simulink model "FYP_Flywheel_Stage5_MODEL_v2"  (R2024a)
settings: Solver=ode45  StartTime=0.0  StopTime=18  RelTol=1e-3
values from neighbouring files (symbols this model uses):
  B = 1.0e-3    (= 0.001)    [FYP_Flywheel_Stage2_build.m]    (also in FYP_Flywheel_Stage3_DCServo_build.m; FYP_Flywheel_Stage4_v2_StableClosedLoop_build.m; FYP_Flywheel_Stage5_COMPLETE_v2.m)
  I_charge = 15    [FYP_Flywheel_Stage5_COMPLETE_v2.m]
  I_discharge = 15    [FYP_Flywheel_Stage5_COMPLETE_v2.m]
  Imax = 18    [FYP_Flywheel_Stage4_v2_StableClosedLoop_build.m]    (also in FYP_Flywheel_Stage5_COMPLETE_v2.m = 20)
  J_total = Jm + Jf    (= 0.51)    [FYP_Flywheel_Stage3_DCServo_build.m]    (also in FYP_Flywheel_Stage4_v2_StableClosedLoop_build.m; FYP_Flywheel_Stage5_COMPLETE_v2.m)
  Jf = 0.50    (= 0.5)    [FYP_Flywheel_Stage3_DCServo_build.m]    (also in FYP_Flywheel_Stage4_v2_StableClosedLoop_build.m; FYP_Flywheel_Stage5_COMPLETE_v2.m)
  Ke = 0.05    [FYP_Flywheel_Stage3_DCServo_build.m]    (also in FYP_Flywheel_Stage4_v2_StableClosedLoop_build.m; FYP_Flywheel_Stage5_COMPLETE_v2.m)
  Kp_current = 1.0    (= 1)    [FYP_Flywheel_Stage4_v2_StableClosedLoop_build.m]    (also in FYP_Flywheel_Stage5_COMPLETE_v2.m)
  Kt = 0.05    [FYP_Flywheel_Stage3_DCServo_build.m]    (also in FYP_Flywheel_Stage4_v2_StableClosedLoop_build.m; FYP_Flywheel_Stage5_COMPLETE_v2.m)
  L = 0.02    [FYP_Flywheel_Stage3_DCServo_build.m]    (also in FYP_Flywheel_Stage4_v2_StableClosedLoop_build.m; FYP_Flywheel_Stage5_COMPLETE_v2.m)
  omega0 = 2*pi*n0/60    (= 314.159265359)    [FYP_Flywheel_Stage1_build.m]    (also in FYP_Flywheel_Stage2_build.m; FYP_Flywheel_Stage3_DCServo_build.m; FYP_Flywheel_Stage4_v2_StableClosedLoop_build.m; FYP_Flywheel_Stage5_COMPLETE_v2.m)
  omega_max = 2*pi*n_max/60    (= 356.047167407)    [FYP_Flywheel_Stage2_build.m]    (also in FYP_Flywheel_Stage5_COMPLETE_v2.m = 329.867228627)
  omega_min = 2*pi*n_min/60    (= 293.215314335)    [FYP_Flywheel_Stage2_build.m]    (also in FYP_Flywheel_Stage5_COMPLETE_v2.m = 298.451302091)
  R = 0.8    [FYP_Flywheel_Stage3_DCServo_build.m]    (also in FYP_Flywheel_Stage4_v2_StableClosedLoop_build.m; FYP_Flywheel_Stage5_COMPLETE_v2.m)
  Tc = 0.05    [FYP_Flywheel_Stage2_build.m]    (also in FYP_Flywheel_Stage3_DCServo_build.m; FYP_Flywheel_Stage4_v2_StableClosedLoop_build.m; FYP_Flywheel_Stage5_COMPLETE_v2.m)
  Vmax = 60    [FYP_Flywheel_Stage4_v2_StableClosedLoop_build.m]    (also in FYP_Flywheel_Stage5_COMPLETE_v2.m)
settings Model: Creator=cheng  LastModifiedBy=cheng

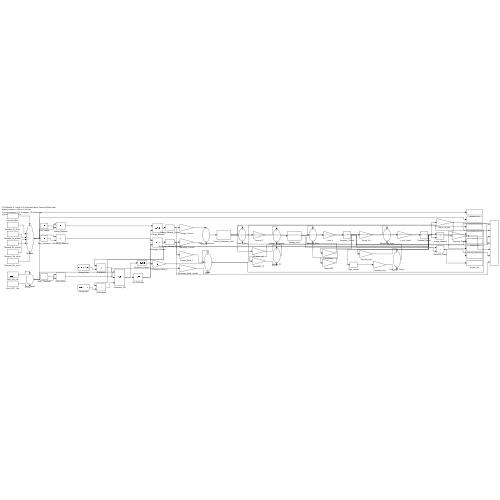
[thumbnail: Simulink's stored preview of the top-level diagram]
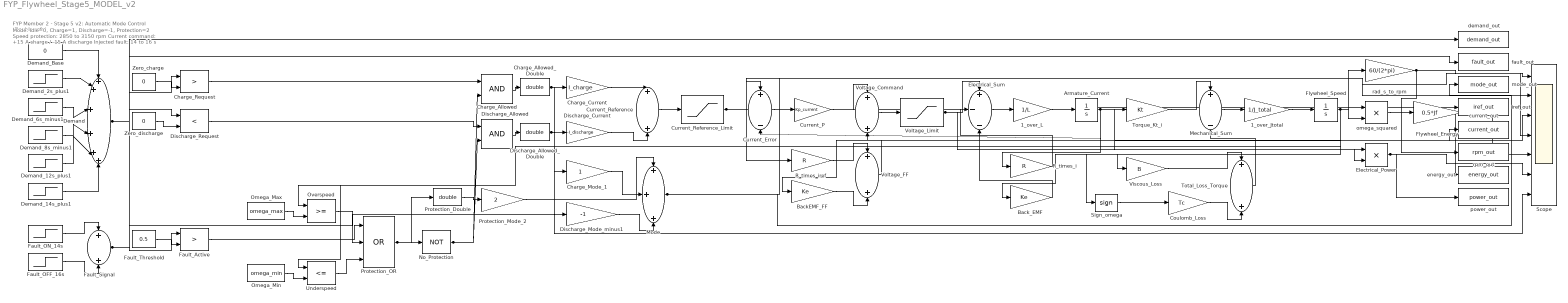
== system FYP_Flywheel_Stage5_MODEL_v2 ==
  note: FYP Member 2 - Stage 5 v2: Automatic Mode Control (Double-safe)
  note: Mode: Idle=0, Charge=1, Discharge=-1, Protection=2
      | Speed protection: 2850 to 3150 rpm
      | Current command: +15 A charge / -15 A discharge
      | Injected fault: 14 to 16 s
  1_over_Jtotal : Gain  Gain=1/J_total
  1_over_L : Gain  Gain=1/L
  Armature_Current : Integrator
  BackEMF_FF : Gain  Gain=Ke
  Back_EMF : Gain  Gain=Ke
  Charge_Allowed : Logic  AllPortsSameDT=off  OutDataTypeStr=boolean
  Charge_Allowed_Double : DataTypeConversion  OutDataTypeStr=double  SaturateOnIntegerOverflow=off  RndMeth=Floor
  Charge_Current : Gain  Gain=I_charge
  Charge_Mode_1 : Gain
  Charge_Request : RelationalOperator  Operator=>  OutDataTypeStr=boolean  RndMeth=Simplest  InputSameDT=off
  Coulomb_Loss : Gain  Gain=Tc
  Current_Error : Sum  Inputs=+-
  Current_P : Gain  Gain=Kp_current
  Current_Reference : Sum
  Current_Reference_Limit : Saturate  UpperLimit=Imax  LowerLimit=-Imax
  Demand : Sum  Inputs=++++++
  Demand_12s_plus1 : Step  Time=12  SampleTime=0
  Demand_14s_plus1 : Step  Time=14  SampleTime=0
  Demand_2s_plus1 : Step  Time=2  SampleTime=0
  Demand_6s_minus1 : Step  Time=6  After=-1  SampleTime=0
  Demand_8s_minus1 : Step  Time=8  After=-1  SampleTime=0
  Demand_Base : Constant  Value=0
  Discharge_Allowed : Logic  AllPortsSameDT=off  OutDataTypeStr=boolean
  Discharge_Allowed_Double : DataTypeConversion  OutDataTypeStr=double  SaturateOnIntegerOverflow=off  RndMeth=Floor
  Discharge_Current : Gain  Gain=-I_discharge
  Discharge_Mode_minus1 : Gain  Gain=-1
  Discharge_Request : RelationalOperator  Operator=<  OutDataTypeStr=boolean  RndMeth=Simplest  InputSameDT=off
  Electrical_Power : Product  Inputs=**
  Electrical_Sum : Sum  Inputs=+--
  Fault_Active : RelationalOperator  Operator=>  OutDataTypeStr=boolean  RndMeth=Simplest  InputSameDT=off
  Fault_OFF_16s : Step  Time=16  After=-1  SampleTime=0
  Fault_ON_14s : Step  Time=14  SampleTime=0
  Fault_Signal : Sum
  Fault_Threshold : Constant  Value=0.5
  Flywheel_Energy : Gain  Gain=0.5*Jf
  Flywheel_Speed : Integrator  InitialCondition=omega0
  Mechanical_Sum : Sum  Inputs=+-
  Mode : Sum  Inputs=+++
  No_Protection : Logic  Operator=NOT  Inputs=1  AllPortsSameDT=off  OutDataTypeStr=boolean
  Omega_Max : Constant  Value=omega_max
  Omega_Min : Constant  Value=omega_min
  Overspeed : RelationalOperator  OutDataTypeStr=boolean  RndMeth=Simplest  InputSameDT=off
  Protection_Double : DataTypeConversion  OutDataTypeStr=double  SaturateOnIntegerOverflow=off  RndMeth=Floor
  Protection_Mode_2 : Gain  Gain=2
  Protection_OR : Logic  Operator=OR  Inputs=3  AllPortsSameDT=off  OutDataTypeStr=boolean
  R_times_i : Gain  Gain=R
  R_times_iref : Gain  Gain=R
  Scope : Scope  NumInputPorts=7
  Sign_omega : Signum
  Torque_Kt_i : Gain  Gain=Kt
  Total_Loss_Torque : Sum
  Underspeed : RelationalOperator  Operator=<=  OutDataTypeStr=boolean  RndMeth=Simplest  InputSameDT=off
  Viscous_Loss : Gain  Gain=B
  Voltage_Command : Sum
  Voltage_FF : Sum
  Voltage_Limit : Saturate  UpperLimit=Vmax  LowerLimit=-Vmax
  Zero_charge : Constant  Value=0
  Zero_discharge : Constant  Value=0
  current_out : ToWorkspace  VariableName=current_out  SaveFormat=Timeseries  SampleTime=-1
  demand_out : ToWorkspace  VariableName=demand_out  SaveFormat=Timeseries  SampleTime=-1
  energy_out : ToWorkspace  VariableName=energy_out  SaveFormat=Timeseries  SampleTime=-1
  fault_out : ToWorkspace  VariableName=fault_out  SaveFormat=Timeseries  SampleTime=-1
  iref_out : ToWorkspace  VariableName=iref_out  SaveFormat=Timeseries  SampleTime=-1
  mode_out : ToWorkspace  VariableName=mode_out  SaveFormat=Timeseries  SampleTime=-1
  omega_squared : Product  Inputs=**
  power_out : ToWorkspace  VariableName=power_out  SaveFormat=Timeseries  SampleTime=-1
  rad_s_to_rpm : Gain  Gain=60/(2*pi)
  rpm_out : ToWorkspace  VariableName=rpm_out  SaveFormat=Timeseries  SampleTime=-1
  wires:
  Demand_Base/1 -> Demand/1
  Demand_2s_plus1/1 -> Demand/2
  Demand_6s_minus1/1 -> Demand/3
  Demand_8s_minus1/1 -> Demand/4
  Demand_12s_plus1/1 -> Demand/5
  Demand_14s_plus1/1 -> Demand/6
  Fault_ON_14s/1 -> Fault_Signal/1
  Fault_OFF_16s/1 -> Fault_Signal/2
  Demand/1 -> Charge_Request/1, Discharge_Request/1, demand_out/1
  Zero_charge/1 -> Charge_Request/2
  Zero_discharge/1 -> Discharge_Request/2
  Fault_Signal/1 -> Fault_Active/1, fault_out/1, Scope/7
  Fault_Threshold/1 -> Fault_Active/2
  Flywheel_Speed/1 -> Overspeed/1, Underspeed/1, BackEMF_FF/1, Back_EMF/1, Viscous_Loss/1, Sign_omega/1, rad_s_to_rpm/1, omega_squared/1, omega_squared/2
  Omega_Max/1 -> Overspeed/2
  Omega_Min/1 -> Underspeed/2
  Fault_Active/1 -> Protection_OR/1
  Overspeed/1 -> Protection_OR/2
  Underspeed/1 -> Protection_OR/3
  Protection_OR/1 -> No_Protection/1, Protection_Double/1
  Charge_Request/1 -> Charge_Allowed/1
  No_Protection/1 -> Charge_Allowed/2, Discharge_Allowed/2
  Discharge_Request/1 -> Discharge_Allowed/1
  Charge_Allowed/1 -> Charge_Allowed_Double/1
  Discharge_Allowed/1 -> Discharge_Allowed_Double/1
  Charge_Allowed_Double/1 -> Charge_Current/1, Charge_Mode_1/1
  Discharge_Allowed_Double/1 -> Discharge_Current/1, Discharge_Mode_minus1/1
  Charge_Current/1 -> Current_Reference/1
  Discharge_Current/1 -> Current_Reference/2
  Current_Reference/1 -> Current_Reference_Limit/1
  Protection_Double/1 -> Protection_Mode_2/1
  Protection_Mode_2/1 -> Mode/1
  Charge_Mode_1/1 -> Mode/2
  Discharge_Mode_minus1/1 -> Mode/3
  Current_Reference_Limit/1 -> Current_Error/1, R_times_iref/1, iref_out/1, Scope/2
  Armature_Current/1 -> Current_Error/2, R_times_i/1, Torque_Kt_i/1, Electrical_Power/2, current_out/1, Scope/3
  Current_Error/1 -> Current_P/1
  R_times_iref/1 -> Voltage_FF/1
  BackEMF_FF/1 -> Voltage_FF/2
  Current_P/1 -> Voltage_Command/1
  Voltage_FF/1 -> Voltage_Command/2
  Voltage_Command/1 -> Voltage_Limit/1
  Voltage_Limit/1 -> Electrical_Sum/1, Electrical_Power/1
  Electrical_Sum/1 -> 1_over_L/1
  1_over_L/1 -> Armature_Current/1
  R_times_i/1 -> Electrical_Sum/2
  Back_EMF/1 -> Electrical_Sum/3
  Torque_Kt_i/1 -> Mechanical_Sum/1
  Viscous_Loss/1 -> Total_Loss_Torque/1
  Sign_omega/1 -> Coulomb_Loss/1
  Coulomb_Loss/1 -> Total_Loss_Torque/2
  Total_Loss_Torque/1 -> Mechanical_Sum/2
  Mechanical_Sum/1 -> 1_over_Jtotal/1
  1_over_Jtotal/1 -> Flywheel_Speed/1
  omega_squared/1 -> Flywheel_Energy/1
  Mode/1 -> mode_out/1, Scope/1
  rad_s_to_rpm/1 -> rpm_out/1, Scope/4
  Flywheel_Energy/1 -> energy_out/1, Scope/5
  Electrical_Power/1 -> power_out/1, Scope/6
